simulink model "VCU_M2"  (R2026a)
settings: Solver=FixedStepDiscrete  StopTime=inf  FixedStep=0.0005  EnableMultiTasking=on
libraries: stm32blockslib x8
settings Model: STM32="{\"CANWrite\":[{\"ID\":\"2\"},{\"ID\":\"3\"},{\"ID\":\"4\"}],\"CANRead\":{\"ID\":\"5\"},\"UARTWrite\":{\"ID\":\"6\"},\"AnalogInput\":{\"ID\":\"1\"},\"DigitalPortWrite\":{\"ID\":\"8\"},\"PWMOutput\":{\"ID\":\"7\"}}"  Creator=1011472417  LastModifiedBy=1011472417
settings HardwareCC: ProdLargestAtomicInteger=Long  ProdLargestAtomicFloat=Double  ProdHWDeviceType=ARM Compatible->ARM Cortex-M
settings RTWCC: SystemTargetFile=ert.tlc  HardwareBoard=STM32F1xx Based  TLCOptions=-aInlineSetEventsForThisBaseRateFcn=TLC_FALSE -aSuppressMultiTaskScheduler=TLC_FALSE -aRateBasedStepFcn=1  Toolchain=GNU Tools for STM32  BuildConfiguration=Faster Runs  Description=Embedded Coder
settings ERTTargetCC: ExtModeTransport=3.0  ExtModeStaticAllocSize=2048.0  CodeReplacementLibrary=ARM Cortex-M

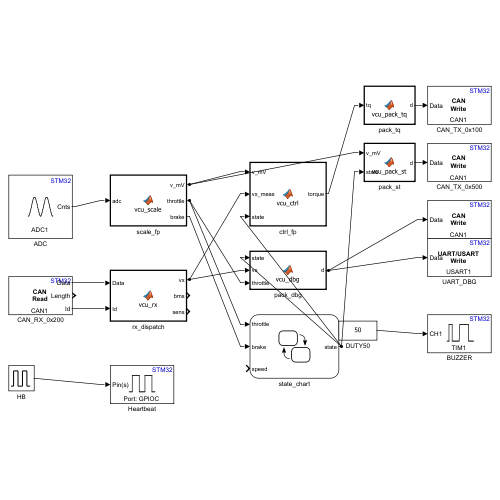
[thumbnail: Simulink's stored preview of the top-level diagram]
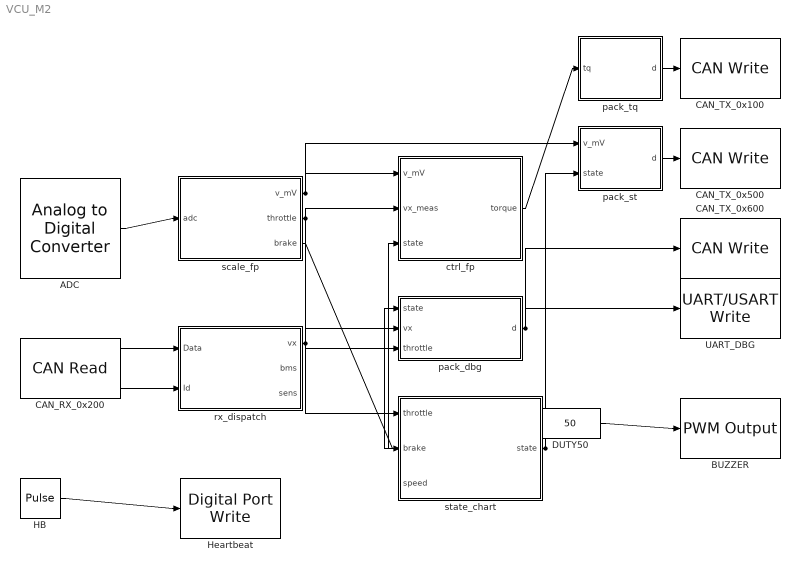
== system VCU_M2 ==
  ADC : stm32blockslib/Analog to Digital Converter  ADCModule=ADC1  ConversionGroup=Regular  TriggerMode=Trigger and read  NumberOfConversions=8  EnableBufferConv=off  BufferLength=1  OutputStatus=off  SampleTime=-1
  BUZZER : stm32blockslib/PWM Output  TimerModule=TIM1  DutycycleUnits=Percentage  EnableChannel1=on  EnableCaptureCompare1Input=off  EnableCaptureCompare1ComplementaryInput=off  EnableOutputCompare1ModeInput=off  EnableChannel2=off  EnableCaptureCompare2Input=off  EnableCaptureCompare2ComplementaryInput=off  EnableOutputCompare2ModeInput=off  EnableChannel3=off  EnableCaptureCompare3Input=off  EnableCaptureCompare3ComplementaryInput=off  EnableOutputCompare3ModeInput=off  EnableChannel4=off  EnableCaptureCompare4Input=off  EnableCaptureCompare4ComplementaryInput=off  EnableOutputCompare4ModeInput=off  EnableChannel5=off  EnableCaptureCompare5Input=off  EnableOutputCompare5ModeInput=off  EnableChannel6=off  EnableCaptureCompare6Input=off  EnableOutputCompare6ModeInput=off  EnableCounterInput=off  EnableMainOutputInput=off  EnableFrequencyInput=off  SetRCAfterCE=off  OutputDirection=off  OutputMainOutputEnableStatus=off  SampleTime=-1  EnableUpdateEvent=off  EnableCaptureCompare1Event=off  EnableCaptureCompare2Event=off  EnableCaptureCompare3Event=off  EnableCaptureCompare4Event=off  EnableTriggerEvent=off  EnableBreakEvent=off  EnableBreakEvent2=off  ProcessorFamily=STM32F4
  CAN_RX_0x200 : stm32blockslib/CAN Read  CANModule=CAN1  BlockMode=Receive  OperationReadMode=Data  OperationWriteMode=Data  OutputTypeReadMode=Unpacked  DataFormatWriteMode=Raw data  ReadSource=FIFO 0  IdentifierTypeVia=Dialog  IdentifierType=Standard (11-bit identifier)  IdentifierVia=Inport  Identifier=100  DataLengthVia=Inport  DataLength=8  OutputIdType=off  TransmitRemoteFrame=off  OutputRemoteFrame=off  OutputTxFifoLevel=off  OutputRxFifoLevel=off  OutputStatus=off  Timeout=0.001  SampleTime=-1
  CAN_TX_0x100 : stm32blockslib/CAN Write  CANModule=CAN1  BlockMode=Transmit  OperationReadMode=Data  OperationWriteMode=Data  OutputTypeReadMode=Unpacked  DataFormatWriteMode=Raw data  ReadSource=FIFO 0  IdentifierTypeVia=Dialog  IdentifierType=Standard (11-bit identifier)  IdentifierVia=Dialog  Identifier=256  DataLengthVia=Dialog  DataLength=8  OutputIdType=off  TransmitRemoteFrame=off  OutputRemoteFrame=off  OutputTxFifoLevel=off  OutputRxFifoLevel=off  OutputStatus=off  Timeout=0.001  SampleTime=-1
  CAN_TX_0x500 : stm32blockslib/CAN Write  CANModule=CAN1  BlockMode=Transmit  OperationReadMode=Data  OperationWriteMode=Data  OutputTypeReadMode=Unpacked  DataFormatWriteMode=Raw data  ReadSource=FIFO 0  IdentifierTypeVia=Dialog  IdentifierType=Standard (11-bit identifier)  IdentifierVia=Dialog  Identifier=1280  DataLengthVia=Dialog  DataLength=8  OutputIdType=off  TransmitRemoteFrame=off  OutputRemoteFrame=off  OutputTxFifoLevel=off  OutputRxFifoLevel=off  OutputStatus=off  Timeout=0.001  SampleTime=-1
  CAN_TX_0x600 : stm32blockslib/CAN Write  CANModule=CAN1  BlockMode=Transmit  OperationReadMode=Data  OperationWriteMode=Data  OutputTypeReadMode=Unpacked  DataFormatWriteMode=Raw data  ReadSource=FIFO 0  IdentifierTypeVia=Dialog  IdentifierType=Standard (11-bit identifier)  IdentifierVia=Dialog  Identifier=1536  DataLengthVia=Dialog  DataLength=8  OutputIdType=off  TransmitRemoteFrame=off  OutputRemoteFrame=off  OutputTxFifoLevel=off  OutputRxFifoLevel=off  OutputStatus=off  Timeout=0.001  SampleTime=-1
  DUTY50 : Constant  Value=50
  HB : DiscretePulseGenerator  PulseType=Time based  PulseWidth=50  SampleTime=0.0005
  Heartbeat : stm32blockslib/Digital Port Write  PortName=GPIOC  PinNumber=[13]  ReadOperation=off  IOAsArray=on  SampleTime=-1
  UART_DBG : stm32blockslib/UART//USART Write  UARTModule=USART1  LengthOfDataToSend=off  BlockingMode=off  BlockingTimeout=0.1  OutputStatus=off
  ctrl_fp : MATLAB Function  TreatAsAtomicUnit=on
  pack_dbg : MATLAB Function  TreatAsAtomicUnit=on
  pack_st : MATLAB Function  TreatAsAtomicUnit=on
  pack_tq : MATLAB Function  TreatAsAtomicUnit=on
  rx_dispatch : MATLAB Function  TreatAsAtomicUnit=on
  scale_fp : MATLAB Function  TreatAsAtomicUnit=on
  state_chart : Stateflow chart  TreatAsAtomicUnit=on
  wires:
  ADC/1 -> scale_fp/1(adc)
  scale_fp/1(v_mV) -> ctrl_fp/1(v_mV), pack_st/1(v_mV)
  CAN_RX_0x200/1 -> rx_dispatch/1(Data)
  CAN_RX_0x200/3 -> rx_dispatch/2(Id)
  rx_dispatch/1(vx) -> ctrl_fp/2(vx_meas), pack_dbg/2(vx)
  state_chart/1(state) -> ctrl_fp/3(state), pack_st/2(state), pack_dbg/1(state)
  scale_fp/2(throttle) -> state_chart/1(throttle), pack_dbg/3(throttle)
  scale_fp/3(brake) -> state_chart/2(brake)
  ctrl_fp/1(torque) -> pack_tq/1(tq)
  pack_tq/1(d) -> CAN_TX_0x100/1
  pack_st/1(d) -> CAN_TX_0x500/1
  pack_dbg/1(d) -> UART_DBG/1, CAN_TX_0x600/1
  DUTY50/1 -> BUZZER/1
  HB/1 -> Heartbeat/1

== matlab function VCU_M2/ctrl_fp ==
  data: v_mV input; torque output; vx_meas input; state input
function torque = vcu_ctrl(v_mV, vx_meas, state)
%#codegen
persistent vx_est
if isempty(vx_est)
    vx_est = int16(0);
end
vx_est = vx_est + int16(0.3*(double(vx_meas)-double(vx_est)));
torque = int16(zeros(4,1));
if state == 1
    b = v_mV(1);
    torque(1)=b; torque(2)=b; torque(3)=b; torque(4)=b;
elseif state == 3
    b = v_mV(3);
    torque(1)=-b; torque(2)=-b; torque(3)=-b; torque(4)=-b;
end
end

== matlab function VCU_M2/scale_fp ==
  data: adc input; v_mV output; throttle output; brake output
function [v_mV, throttle, brake] = vcu_scale(adc)
%#codegen
v_mV = fi(zeros(8,1),1,16,0);
k = fi(3300/4095,1,16,15);
for i = 1:8
    v_mV(i) = fi(adc(i),1,16,0)*k;
end
throttle = v_mV(1);
brake = v_mV(3);
end

== matlab function VCU_M2/pack_tq ==
  data: tq input; d output
function d = vcu_pack_tq(tq)
%#codegen
d = zeros(8,1,'uint8');
for i=1:4
    u = uint16(tq(i));
    d(2*i-1) = uint8(bitshift(u,-8));
    d(2*i)   = uint8(bitand(u,255));
end
end

== matlab function VCU_M2/pack_st ==
  data: v_mV input; d output; state input
function d = vcu_pack_st(v_mV, state)
%#codegen
d = zeros(8,1,'uint8');
d(1) = uint8(state);
for i=1:3
    u = uint16(v_mV(i));
    d(2*i) = uint8(bitshift(u,-8));
    d(2*i+1) = uint8(bitand(u,255));
end
end

== matlab function VCU_M2/rx_dispatch ==
  data: Data input; vx output; Id input; bms output; sens output
function [vx, bms, sens] = vcu_rx(Data, Id)
%#codegen
vx = int16(0); bms = int16(0); sens = int16(0);
if Id == uint32(512)
    vx = int16(bitshift(uint16(Data(1)),8) + uint16(Data(2)));
elseif Id == uint32(768)
    bms = int16(bitshift(uint16(Data(1)),8) + uint16(Data(2)));
elseif Id == uint32(1024)
    sens = int16(bitshift(uint16(Data(1)),8) + uint16(Data(2)));
end
end

== matlab function VCU_M2/pack_dbg ==
  data: state input; d output; vx input; throttle input
function d = vcu_dbg(state, vx, throttle)
%#codegen
d = zeros(8,1,'uint8');
d(1)=uint8(state);
u=uint16(vx); d(2)=uint8(bitshift(u,-8)); d(3)=uint8(bitand(u,255));
u=uint16(throttle); d(4)=uint8(bitshift(u,-8)); d(5)=uint8(bitand(u,255));
end

== stateflow chart VCU_M2/state_chart ==
  state Start
  state Drive
  state Brake
  Brake -> Start [order 2] : [speed <= 0 && throttle <= 50] {state = uint8(0);}
  Drive -> Start [order 1] : [throttle <= 50 && speed <= 0] {state = uint8(0);}
  (default) -> Start : {state = uint8(0);}
  Brake -> Drive [order 1] : [brake <= 50 && throttle > 50] {state = uint8(1);}
  Start -> Drive : [throttle > 50] {state = uint8(1);}
  Drive -> Brake [order 2] : [brake > 50] {state = uint8(3);}
  data: throttle input int16; brake input int16; speed input int16; state output uint8
